simulink model "ball_on_beam_sim"  (R2018a)
settings: Solver=ode45  StartTime=0.0  StopTime=10000  MaxStep=0.1  RelTol=1e-3
undefined symbols (not defined in the file or in its folder): ball_on_beam_animation
libraries: simulink x2
settings Model: Creator=canla  LastModifiedBy=canla
settings OptimizationCC: LifeSpan=inf

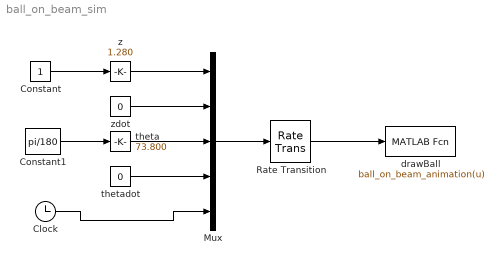
== system ball_on_beam_sim ==
  Clock : Clock
  Constant : Constant
  Constant1 : Constant  Value=pi/180
  Mux : Mux  Inputs=5
  Rate Transition : RateTransition  OutPortSampleTimeMultiple=P.t_plot  OutPortSampleTime=P.t_plot
  drawBall : MATLABFcn  MATLABFcn=ball_on_beam_animation(u)  OutputDimensions=0
  theta : simulink/Math Operations/Slider Gain  gain=73.800  low=0  high=90
  "thetadot " : Constant  Value=0
  z : simulink/Math Operations/Slider Gain  gain=1.280  low=0.5  high=2.5
  zdot : Constant  Value=0
  wires:
  zdot/1 -> Mux/2
  "thetadot "/1 -> Mux/4
  z/1 -> Mux/1
  Constant/1 -> z/1
  theta/1 -> Mux/3
  Constant1/1 -> theta/1
  Clock/1 -> Mux/5
  Mux/1 -> Rate Transition/1
  Rate Transition/1 -> drawBall/1
